simulink model "gm_UZ_EnDat"  (R2023b)
settings: Solver=FixedStepDiscrete  StartTime=0  StopTime=0.002  RelTol=1e-3
model workspace (MAT data in the model file):
  Select = 0
libraries: hdlsllib x314, hdlmdlgenlib x10, simulink x7, simulink_extras x3
(part 5 of 7)

== system gm_UZ_EnDat/UZ_ENDAT/CLKCNTER_ACT/Positional_Counter/Increment Stored Integer ==
  u : Inport  OutDataTypeStr=uint32
  FixPt Constant : Constant  OutDataTypeStr=uint32  SampleTime=-1
  FixPt Data Type Duplicate : DataTypeDuplicate  DisableCoverage=on  NumInputPorts=3
  FixPt Gateway In : DataTypeConversion  OutDataTypeStr=fixdt(0,32,0)
  FixPt Sum1 : Sum  OutDataTypeStr=uint32  AccumDataTypeStr=uint32
  sigspec : SignalSpecification  OutDataTypeStr=uint32  Dimensions=1
  y : Outport  InitialOutput=0
  wires:
  sigspec/1 -> FixPt Gateway In/1
  FixPt Sum1/1 -> y/1, FixPt Data Type Duplicate/1
  FixPt Gateway In/1 -> FixPt Data Type Duplicate/3, FixPt Sum1/2
  FixPt Constant/1 -> sigspec/1
  u/1 -> FixPt Data Type Duplicate/2, FixPt Sum1/1

== system gm_UZ_EnDat/UZ_ENDAT/CLKCNTER_NOSTOP/Positional_Counter/Increment Stored Integer ==
  u : Inport  OutDataTypeStr=uint32
  FixPt Constant : Constant  OutDataTypeStr=uint32  SampleTime=-1
  FixPt Data Type Duplicate : DataTypeDuplicate  DisableCoverage=on  NumInputPorts=3
  FixPt Gateway In : DataTypeConversion  OutDataTypeStr=fixdt(0,32,0)
  FixPt Sum1 : Sum  OutDataTypeStr=uint32  AccumDataTypeStr=uint32
  sigspec : SignalSpecification  OutDataTypeStr=uint32  Dimensions=1
  y : Outport  InitialOutput=0
  wires:
  u/1 -> FixPt Sum1/1, FixPt Data Type Duplicate/2
  FixPt Constant/1 -> sigspec/1
  FixPt Gateway In/1 -> FixPt Sum1/2, FixPt Data Type Duplicate/3
  FixPt Sum1/1 -> FixPt Data Type Duplicate/1, y/1
  sigspec/1 -> FixPt Gateway In/1

== system gm_UZ_EnDat/UZ_ENDAT/CRC_Check/DFF1/JKFF ==
  SET : Inport  OutDataTypeStr=boolean  PortDimensions=1  SampleTime=1e-08
  CLK : Inport  Port=2  OutDataTypeStr=boolean  PortDimensions=1  SampleTime=1e-08
  J : Inport  Port=3  OutDataTypeStr=boolean  PortDimensions=1  SampleTime=1e-08
  RST : Inport  Port=4  OutDataTypeStr=boolean  PortDimensions=1  SampleTime=1e-08
  K : Inport  Port=5  OutDataTypeStr=boolean  PortDimensions=1  SampleTime=1e-08
  AND : Logic  Inputs=4  AllPortsSameDT=off  OutDataTypeStr=boolean  SampleTime=1e-08
  AND1 : Logic  Inputs=4  AllPortsSameDT=off  OutDataTypeStr=boolean  SampleTime=1e-08
  AND{2..5} (4 alike) : Logic  AllPortsSameDT=off  OutDataTypeStr=boolean  SampleTime=1e-08
  Delay{,1..3} (4 alike) : Delay  DelayLength=double(1)  InitialCondition=0  SampleTime=1e-08
  NOR : Logic  Operator=NOR  Inputs=4  AllPortsSameDT=off  OutDataTypeStr=boolean  SampleTime=1e-08
  NOR1 : Logic  Operator=NOR  Inputs=4  AllPortsSameDT=off  OutDataTypeStr=boolean  SampleTime=1e-08
  NOR2 : Logic  Operator=NOR  AllPortsSameDT=off  OutDataTypeStr=boolean  SampleTime=1e-08
  NOR3 : Logic  Operator=NAND  AllPortsSameDT=off  OutDataTypeStr=boolean  SampleTime=1e-08
  NOR4 : Logic  Operator=NOR  AllPortsSameDT=off  OutDataTypeStr=boolean  SampleTime=1e-08
  NOR5 : Logic  Operator=NAND  AllPortsSameDT=off  OutDataTypeStr=boolean  SampleTime=1e-08
  NOT : Logic  Operator=NOT  Inputs=1  AllPortsSameDT=off  OutDataTypeStr=boolean  SampleTime=1e-08
  NOT1 : Logic  Operator=NOT  Inputs=1  AllPortsSameDT=off  OutDataTypeStr=boolean  SampleTime=1e-08
  OR : Logic  Operator=OR  Inputs=3  AllPortsSameDT=off  OutDataTypeStr=boolean  SampleTime=1e-08
  OQ : Outport  SampleTime=1e-08
  NOQ : Outport  Port=2  SampleTime=1e-08
  wires:
  SET/1 -> NOR2/1, NOR/1
  CLK/1 -> OR/2, NOT/1, AND5/1, AND4/2
  J/1 -> OR/1, AND/2
  RST/1 -> NOR1/4, NOR4/2
  K/1 -> OR/3, AND1/3
  Delay2/1 -> NOQ/1, AND2/2, NOR3/2, AND/1
  Delay3/1 -> OQ/1, AND1/4, AND3/1, NOR5/1
  NOT/1 -> AND1/2, AND/3
  NOT1/1 -> AND2/1, AND3/2
  OR/1 -> NOT1/1, AND1/1, AND/4
  Delay/1 -> NOR1/1, AND4/1
  Delay1/1 -> AND5/2, NOR/4
  NOR/1 -> Delay/1
  AND3/1 -> NOR/3
  AND/1 -> NOR/2
  NOR5/1 -> Delay2/1
  AND4/1 -> NOR4/1
  NOR4/1 -> NOR5/2
  NOR1/1 -> Delay1/1
  AND1/1 -> NOR1/3
  AND2/1 -> NOR1/2
  NOR3/1 -> Delay3/1
  AND5/1 -> NOR2/2
  NOR2/1 -> NOR3/1

== system gm_UZ_EnDat/UZ_ENDAT/CRC_Check/DFF2/JKFF ==
  SET : Inport  OutDataTypeStr=boolean  PortDimensions=1  SampleTime=1e-08
  CLK : Inport  Port=2  OutDataTypeStr=boolean  PortDimensions=1  SampleTime=1e-08
  J : Inport  Port=3  OutDataTypeStr=boolean  PortDimensions=1  SampleTime=1e-08
  RST : Inport  Port=4  OutDataTypeStr=boolean  PortDimensions=1  SampleTime=1e-08
  K : Inport  Port=5  OutDataTypeStr=boolean  PortDimensions=1  SampleTime=1e-08
  AND : Logic  Inputs=4  AllPortsSameDT=off  OutDataTypeStr=boolean  SampleTime=1e-08
  AND1 : Logic  Inputs=4  AllPortsSameDT=off  OutDataTypeStr=boolean  SampleTime=1e-08
  AND{2..5} (4 alike) : Logic  AllPortsSameDT=off  OutDataTypeStr=boolean  SampleTime=1e-08
  Delay{,1..3} (4 alike) : Delay  DelayLength=double(1)  InitialCondition=0  SampleTime=1e-08
  NOR : Logic  Operator=NOR  Inputs=4  AllPortsSameDT=off  OutDataTypeStr=boolean  SampleTime=1e-08
  NOR1 : Logic  Operator=NOR  Inputs=4  AllPortsSameDT=off  OutDataTypeStr=boolean  SampleTime=1e-08
  NOR2 : Logic  Operator=NOR  AllPortsSameDT=off  OutDataTypeStr=boolean  SampleTime=1e-08
  NOR3 : Logic  Operator=NAND  AllPortsSameDT=off  OutDataTypeStr=boolean  SampleTime=1e-08
  NOR4 : Logic  Operator=NOR  AllPortsSameDT=off  OutDataTypeStr=boolean  SampleTime=1e-08
  NOR5 : Logic  Operator=NAND  AllPortsSameDT=off  OutDataTypeStr=boolean  SampleTime=1e-08
  NOT : Logic  Operator=NOT  Inputs=1  AllPortsSameDT=off  OutDataTypeStr=boolean  SampleTime=1e-08
  NOT1 : Logic  Operator=NOT  Inputs=1  AllPortsSameDT=off  OutDataTypeStr=boolean  SampleTime=1e-08
  OR : Logic  Operator=OR  Inputs=3  AllPortsSameDT=off  OutDataTypeStr=boolean  SampleTime=1e-08
  OQ : Outport  SampleTime=1e-08
  NOQ : Outport  Port=2  SampleTime=1e-08
  wires:
  NOR2/1 -> NOR3/1
  AND5/1 -> NOR2/2
  NOR3/1 -> Delay3/1
  AND2/1 -> NOR1/2
  AND1/1 -> NOR1/3
  NOR1/1 -> Delay1/1
  NOR4/1 -> NOR5/2
  AND4/1 -> NOR4/1
  NOR5/1 -> Delay2/1
  AND/1 -> NOR/2
  AND3/1 -> NOR/3
  NOR/1 -> Delay/1
  Delay1/1 -> NOR/4, AND5/2
  Delay/1 -> AND4/1, NOR1/1
  OR/1 -> AND/4, AND1/1, NOT1/1
  NOT1/1 -> AND3/2, AND2/1
  NOT/1 -> AND/3, AND1/2
  Delay3/1 -> NOR5/1, AND3/1, AND1/4, OQ/1
  Delay2/1 -> AND/1, NOR3/2, AND2/2, NOQ/1
  K/1 -> AND1/3, OR/3
  RST/1 -> NOR4/2, NOR1/4
  J/1 -> AND/2, OR/1
  CLK/1 -> AND4/2, AND5/1, NOT/1, OR/2
  SET/1 -> NOR/1, NOR2/1

== system gm_UZ_EnDat/UZ_ENDAT/CRC_Check/DFF3/JKFF ==
  SET : Inport  OutDataTypeStr=boolean  PortDimensions=1  SampleTime=1e-08
  CLK : Inport  Port=2  OutDataTypeStr=boolean  PortDimensions=1  SampleTime=1e-08
  J : Inport  Port=3  OutDataTypeStr=boolean  PortDimensions=1  SampleTime=1e-08
  RST : Inport  Port=4  OutDataTypeStr=boolean  PortDimensions=1  SampleTime=1e-08
  K : Inport  Port=5  OutDataTypeStr=boolean  PortDimensions=1  SampleTime=1e-08
  AND : Logic  Inputs=4  AllPortsSameDT=off  OutDataTypeStr=boolean  SampleTime=1e-08
  AND1 : Logic  Inputs=4  AllPortsSameDT=off  OutDataTypeStr=boolean  SampleTime=1e-08
  AND{2..5} (4 alike) : Logic  AllPortsSameDT=off  OutDataTypeStr=boolean  SampleTime=1e-08
  Delay{,1..3} (4 alike) : Delay  DelayLength=double(1)  InitialCondition=0  SampleTime=1e-08
  NOR : Logic  Operator=NOR  Inputs=4  AllPortsSameDT=off  OutDataTypeStr=boolean  SampleTime=1e-08
  NOR1 : Logic  Operator=NOR  Inputs=4  AllPortsSameDT=off  OutDataTypeStr=boolean  SampleTime=1e-08
  NOR2 : Logic  Operator=NOR  AllPortsSameDT=off  OutDataTypeStr=boolean  SampleTime=1e-08
  NOR3 : Logic  Operator=NAND  AllPortsSameDT=off  OutDataTypeStr=boolean  SampleTime=1e-08
  NOR4 : Logic  Operator=NOR  AllPortsSameDT=off  OutDataTypeStr=boolean  SampleTime=1e-08
  NOR5 : Logic  Operator=NAND  AllPortsSameDT=off  OutDataTypeStr=boolean  SampleTime=1e-08
  NOT : Logic  Operator=NOT  Inputs=1  AllPortsSameDT=off  OutDataTypeStr=boolean  SampleTime=1e-08
  NOT1 : Logic  Operator=NOT  Inputs=1  AllPortsSameDT=off  OutDataTypeStr=boolean  SampleTime=1e-08
  OR : Logic  Operator=OR  Inputs=3  AllPortsSameDT=off  OutDataTypeStr=boolean  SampleTime=1e-08
  OQ : Outport  SampleTime=1e-08
  NOQ : Outport  Port=2  SampleTime=1e-08
  wires:
  NOR2/1 -> NOR3/1
  AND5/1 -> NOR2/2
  NOR3/1 -> Delay3/1
  AND2/1 -> NOR1/2
  AND1/1 -> NOR1/3
  NOR1/1 -> Delay1/1
  NOR4/1 -> NOR5/2
  AND4/1 -> NOR4/1
  NOR5/1 -> Delay2/1
  AND/1 -> NOR/2
  AND3/1 -> NOR/3
  NOR/1 -> Delay/1
  Delay1/1 -> NOR/4, AND5/2
  Delay/1 -> AND4/1, NOR1/1
  OR/1 -> AND/4, AND1/1, NOT1/1
  NOT1/1 -> AND3/2, AND2/1
  NOT/1 -> AND/3, AND1/2
  Delay3/1 -> NOR5/1, AND3/1, AND1/4, OQ/1
  Delay2/1 -> AND/1, NOR3/2, AND2/2, NOQ/1
  K/1 -> AND1/3, OR/3
  RST/1 -> NOR4/2, NOR1/4
  J/1 -> AND/2, OR/1
  CLK/1 -> AND4/2, AND5/1, NOT/1, OR/2
  SET/1 -> NOR/1, NOR2/1

== system gm_UZ_EnDat/UZ_ENDAT/CRC_Check/DFF4/JKFF ==
  SET : Inport  OutDataTypeStr=boolean  PortDimensions=1  SampleTime=1e-08
  CLK : Inport  Port=2  OutDataTypeStr=boolean  PortDimensions=1  SampleTime=1e-08
  J : Inport  Port=3  OutDataTypeStr=boolean  PortDimensions=1  SampleTime=1e-08
  RST : Inport  Port=4  OutDataTypeStr=boolean  PortDimensions=1  SampleTime=1e-08
  K : Inport  Port=5  OutDataTypeStr=boolean  PortDimensions=1  SampleTime=1e-08
  AND : Logic  Inputs=4  AllPortsSameDT=off  OutDataTypeStr=boolean  SampleTime=1e-08
  AND1 : Logic  Inputs=4  AllPortsSameDT=off  OutDataTypeStr=boolean  SampleTime=1e-08
  AND{2..5} (4 alike) : Logic  AllPortsSameDT=off  OutDataTypeStr=boolean  SampleTime=1e-08
  Delay{,1..3} (4 alike) : Delay  DelayLength=double(1)  InitialCondition=0  SampleTime=1e-08
  NOR : Logic  Operator=NOR  Inputs=4  AllPortsSameDT=off  OutDataTypeStr=boolean  SampleTime=1e-08
  NOR1 : Logic  Operator=NOR  Inputs=4  AllPortsSameDT=off  OutDataTypeStr=boolean  SampleTime=1e-08
  NOR2 : Logic  Operator=NOR  AllPortsSameDT=off  OutDataTypeStr=boolean  SampleTime=1e-08
  NOR3 : Logic  Operator=NAND  AllPortsSameDT=off  OutDataTypeStr=boolean  SampleTime=1e-08
  NOR4 : Logic  Operator=NOR  AllPortsSameDT=off  OutDataTypeStr=boolean  SampleTime=1e-08
  NOR5 : Logic  Operator=NAND  AllPortsSameDT=off  OutDataTypeStr=boolean  SampleTime=1e-08
  NOT : Logic  Operator=NOT  Inputs=1  AllPortsSameDT=off  OutDataTypeStr=boolean  SampleTime=1e-08
  NOT1 : Logic  Operator=NOT  Inputs=1  AllPortsSameDT=off  OutDataTypeStr=boolean  SampleTime=1e-08
  OR : Logic  Operator=OR  Inputs=3  AllPortsSameDT=off  OutDataTypeStr=boolean  SampleTime=1e-08
  OQ : Outport  SampleTime=1e-08
  NOQ : Outport  Port=2  SampleTime=1e-08
  wires:
  NOR2/1 -> NOR3/1
  AND5/1 -> NOR2/2
  NOR3/1 -> Delay3/1
  AND2/1 -> NOR1/2
  AND1/1 -> NOR1/3
  NOR1/1 -> Delay1/1
  NOR4/1 -> NOR5/2
  AND4/1 -> NOR4/1
  NOR5/1 -> Delay2/1
  AND/1 -> NOR/2
  AND3/1 -> NOR/3
  NOR/1 -> Delay/1
  Delay1/1 -> NOR/4, AND5/2
  Delay/1 -> AND4/1, NOR1/1
  OR/1 -> AND/4, AND1/1, NOT1/1
  NOT1/1 -> AND3/2, AND2/1
  NOT/1 -> AND/3, AND1/2
  Delay3/1 -> NOR5/1, AND3/1, AND1/4, OQ/1
  Delay2/1 -> AND/1, NOR3/2, AND2/2, NOQ/1
  K/1 -> AND1/3, OR/3
  RST/1 -> NOR4/2, NOR1/4
  J/1 -> AND/2, OR/1
  CLK/1 -> AND4/2, AND5/1, NOT/1, OR/2
  SET/1 -> NOR/1, NOR2/1

== system gm_UZ_EnDat/UZ_ENDAT/CRC_Check/DFF5/JKFF ==
  SET : Inport  OutDataTypeStr=boolean  PortDimensions=1  SampleTime=1e-08
  CLK : Inport  Port=2  OutDataTypeStr=boolean  PortDimensions=1  SampleTime=1e-08
  J : Inport  Port=3  OutDataTypeStr=boolean  PortDimensions=1  SampleTime=1e-08
  RST : Inport  Port=4  OutDataTypeStr=boolean  PortDimensions=1  SampleTime=1e-08
  K : Inport  Port=5  OutDataTypeStr=boolean  PortDimensions=1  SampleTime=1e-08
  AND : Logic  Inputs=4  AllPortsSameDT=off  OutDataTypeStr=boolean  SampleTime=1e-08
  AND1 : Logic  Inputs=4  AllPortsSameDT=off  OutDataTypeStr=boolean  SampleTime=1e-08
  AND{2..5} (4 alike) : Logic  AllPortsSameDT=off  OutDataTypeStr=boolean  SampleTime=1e-08
  Delay{,1..3} (4 alike) : Delay  DelayLength=double(1)  InitialCondition=0  SampleTime=1e-08
  NOR : Logic  Operator=NOR  Inputs=4  AllPortsSameDT=off  OutDataTypeStr=boolean  SampleTime=1e-08
  NOR1 : Logic  Operator=NOR  Inputs=4  AllPortsSameDT=off  OutDataTypeStr=boolean  SampleTime=1e-08
  NOR2 : Logic  Operator=NOR  AllPortsSameDT=off  OutDataTypeStr=boolean  SampleTime=1e-08
  NOR3 : Logic  Operator=NAND  AllPortsSameDT=off  OutDataTypeStr=boolean  SampleTime=1e-08
  NOR4 : Logic  Operator=NOR  AllPortsSameDT=off  OutDataTypeStr=boolean  SampleTime=1e-08
  NOR5 : Logic  Operator=NAND  AllPortsSameDT=off  OutDataTypeStr=boolean  SampleTime=1e-08
  NOT : Logic  Operator=NOT  Inputs=1  AllPortsSameDT=off  OutDataTypeStr=boolean  SampleTime=1e-08
  NOT1 : Logic  Operator=NOT  Inputs=1  AllPortsSameDT=off  OutDataTypeStr=boolean  SampleTime=1e-08
  OR : Logic  Operator=OR  Inputs=3  AllPortsSameDT=off  OutDataTypeStr=boolean  SampleTime=1e-08
  OQ : Outport  SampleTime=1e-08
  NOQ : Outport  Port=2  SampleTime=1e-08
  wires:
  NOR2/1 -> NOR3/1
  AND5/1 -> NOR2/2
  NOR3/1 -> Delay3/1
  AND2/1 -> NOR1/2
  AND1/1 -> NOR1/3
  NOR1/1 -> Delay1/1
  NOR4/1 -> NOR5/2
  AND4/1 -> NOR4/1
  NOR5/1 -> Delay2/1
  AND/1 -> NOR/2
  AND3/1 -> NOR/3
  NOR/1 -> Delay/1
  Delay1/1 -> NOR/4, AND5/2
  Delay/1 -> AND4/1, NOR1/1
  OR/1 -> AND/4, AND1/1, NOT1/1
  NOT1/1 -> AND3/2, AND2/1
  NOT/1 -> AND/3, AND1/2
  Delay3/1 -> NOR5/1, AND3/1, AND1/4, OQ/1
  Delay2/1 -> AND/1, NOR3/2, AND2/2, NOQ/1
  K/1 -> AND1/3, OR/3
  RST/1 -> NOR4/2, NOR1/4
  J/1 -> AND/2, OR/1
  CLK/1 -> AND4/2, AND5/1, NOT/1, OR/2
  SET/1 -> NOR/1, NOR2/1

== system gm_UZ_EnDat/UZ_ENDAT/INITIALOFF/CLKCNTER_FAST/Positional_Counter ==
  valueout : Inport  OutDataTypeStr=uint32  PortDimensions=1
  Trigger : TriggerPort  TriggerType=either  VariantControl=(inherit)  InitialTriggerSignalState=zero  PortDimensions=1  OutDataTypeStr=boolean
  Add : Sum  OutDataTypeStr=fixdt(0, 33, 0)  AccumDataTypeStr=fixdt(0, 33, 0)
  Add_out_dtc : DataTypeConversion  OutDataTypeStr=uint32  RndMeth=Simplest
  Constant : Constant  OutDataTypeStr=uint32  SampleTime=-1
  divider : Outport  InitialOutput=0
  wires:
  valueout/1 -> Add/1
  Add_out_dtc/1 -> divider/1
  Constant/1 -> Add/2
  Add/1 -> Add_out_dtc/1

== system gm_UZ_EnDat/UZ_ENDAT/INITIALOFF/Subsystem6/Compare To Constant ==
  u : Inport  OutDataTypeStr=uint16  SampleTime=1e-08
  Compare : RelationalOperator  Operator=<  OutDataTypeStr=boolean  SampleTime=1e-08
  Constant : Constant  Value=100  OutDataTypeStr=uint16  SampleTime=1e-08
  y : Outport  SampleTime=1e-08
  wires:
  u/1 -> Compare/1
  Compare/1 -> y/1
  Constant/1 -> Compare/2

== system gm_UZ_EnDat/UZ_ENDAT/ManualSerialize/Storage1/Compare To Zero ==
  u : Inport  OutDataTypeStr=fixdt(0, 64, 0)  SampleTime=1e-08
  Compare : RelationalOperator  Operator=>  OutDataTypeStr=boolean  SampleTime=1e-08
  Constant : Constant  Value="fi(0,0,64,0,\"hex\",\"0000000000000000\")"  OutDataTypeStr=fixdt(0, 64, 0)  SampleTime=1e-08
  y : Outport  SampleTime=1e-08
  wires:
  u/1 -> Compare/1
  Compare/1 -> y/1
  Constant/1 -> Compare/2

== system gm_UZ_EnDat/UZ_ENDAT/ManualSerialize/Subsystem/Detect Increase ==
  note: U(k)
  note: Edge
  U : Inport  OutDataTypeStr=boolean  SampleTime=1e-08
  FixPt Relational Operator : RelationalOperator  Operator=>  OutDataTypeStr=boolean  SampleTime=1e-08  InputSameDT=off
  rd_0 : Delay  DelayLength=double(1)  InitialCondition=0  SampleTime=1e-08
  t : hdlmdlgenlib/Buffer
  Y : Outport  SampleTime=1e-08
  wires:
  U/1 -> t/1, FixPt Relational Operator/1
  t/1 -> rd_0/1
  FixPt Relational Operator/1 -> Y/1
  rd_0/1 -> FixPt Relational Operator/2

== system gm_UZ_EnDat/UZ_ENDAT/ManualSerialize/padder/nibblepadding1 ==
  in : Inport  OutDataTypeStr=fixdt(0, 64, 0)  PortDimensions=1  SampleTime=1e-08
  padding1 : Subsystem
  padding2 : Subsystem
  padding3 : Subsystem
  out : Outport  SampleTime=1e-08
  wires:
  in/1 -> padding3/1(in)
  padding1/1(out) -> out/1
  padding2/1(out) -> padding1/1(in)
  padding3/1(out) -> padding2/1(in)

== system gm_UZ_EnDat/UZ_ENDAT/ManualSerialize/padder/nibblepadding10 ==
  in : Inport  OutDataTypeStr=fixdt(0, 64, 0)  PortDimensions=1  SampleTime=1e-08
  padding1 : Subsystem
  padding2 : Subsystem
  padding3 : Subsystem
  out : Outport  SampleTime=1e-08
  wires:
  padding3/1(out) -> padding2/1(in)
  padding2/1(out) -> padding1/1(in)
  padding1/1(out) -> out/1
  in/1 -> padding3/1(in)

== system gm_UZ_EnDat/UZ_ENDAT/ManualSerialize/padder/nibblepadding11 ==
  in : Inport  OutDataTypeStr=fixdt(0, 64, 0)  PortDimensions=1  SampleTime=1e-08
  padding1 : Subsystem
  padding2 : Subsystem
  padding3 : Subsystem
  out : Outport  SampleTime=1e-08
  wires:
  padding3/1(out) -> padding2/1(in)
  padding2/1(out) -> padding1/1(in)
  padding1/1(out) -> out/1
  in/1 -> padding3/1(in)

== system gm_UZ_EnDat/UZ_ENDAT/ManualSerialize/padder/nibblepadding12 ==
  in : Inport  OutDataTypeStr=fixdt(0, 64, 0)  PortDimensions=1  SampleTime=1e-08
  padding1 : Subsystem
  padding2 : Subsystem
  padding3 : Subsystem
  out : Outport  SampleTime=1e-08
  wires:
  padding3/1(out) -> padding2/1(in)
  padding2/1(out) -> padding1/1(in)
  padding1/1(out) -> out/1
  in/1 -> padding3/1(in)

== system gm_UZ_EnDat/UZ_ENDAT/ManualSerialize/padder/nibblepadding13 ==
  in : Inport  OutDataTypeStr=fixdt(0, 64, 0)  PortDimensions=1  SampleTime=1e-08
  padding1 : Subsystem
  padding2 : Subsystem
  padding3 : Subsystem
  out : Outport  SampleTime=1e-08
  wires:
  padding3/1(out) -> padding2/1(in)
  padding2/1(out) -> padding1/1(in)
  padding1/1(out) -> out/1
  in/1 -> padding3/1(in)

== system gm_UZ_EnDat/UZ_ENDAT/ManualSerialize/padder/nibblepadding14 ==
  in : Inport  OutDataTypeStr=fixdt(0, 64, 0)  PortDimensions=1  SampleTime=1e-08
  padding1 : Subsystem
  padding2 : Subsystem
  padding3 : Subsystem
  out : Outport  SampleTime=1e-08
  wires:
  padding3/1(out) -> padding2/1(in)
  padding2/1(out) -> padding1/1(in)
  padding1/1(out) -> out/1
  in/1 -> padding3/1(in)

== system gm_UZ_EnDat/UZ_ENDAT/ManualSerialize/padder/nibblepadding15 ==
  in : Inport  OutDataTypeStr=fixdt(0, 64, 0)  PortDimensions=1  SampleTime=1e-08
  padding1 : Subsystem
  padding2 : Subsystem
  padding3 : Subsystem
  out : Outport  SampleTime=1e-08
  wires:
  padding3/1(out) -> padding2/1(in)
  padding2/1(out) -> padding1/1(in)
  padding1/1(out) -> out/1
  in/1 -> padding3/1(in)

== system gm_UZ_EnDat/UZ_ENDAT/ManualSerialize/padder/nibblepadding16 ==
  in : Inport  OutDataTypeStr=fixdt(0, 64, 0)  PortDimensions=1  SampleTime=1e-08
  padding1 : Subsystem
  padding2 : Subsystem
  padding3 : Subsystem
  out : Outport  SampleTime=1e-08
  wires:
  padding3/1(out) -> padding2/1(in)
  padding2/1(out) -> padding1/1(in)
  padding1/1(out) -> out/1
  in/1 -> padding3/1(in)

== system gm_UZ_EnDat/UZ_ENDAT/ManualSerialize/padder/nibblepadding17 ==
  in : Inport  OutDataTypeStr=fixdt(0, 64, 0)  PortDimensions=1  SampleTime=1e-08
  padding1 : Subsystem
  padding2 : Subsystem
  padding3 : Subsystem
  out : Outport  SampleTime=1e-08
  wires:
  padding3/1(out) -> padding2/1(in)
  padding2/1(out) -> padding1/1(in)
  padding1/1(out) -> out/1
  in/1 -> padding3/1(in)

== system gm_UZ_EnDat/UZ_ENDAT/ManualSerialize/padder/nibblepadding18 ==
  in : Inport  OutDataTypeStr=fixdt(0, 64, 0)  PortDimensions=1  SampleTime=1e-08
  padding1 : Subsystem
  padding2 : Subsystem
  padding3 : Subsystem
  out : Outport  SampleTime=1e-08
  wires:
  padding3/1(out) -> padding2/1(in)
  padding2/1(out) -> padding1/1(in)
  padding1/1(out) -> out/1
  in/1 -> padding3/1(in)

== system gm_UZ_EnDat/UZ_ENDAT/ManualSerialize/padder/nibblepadding19 ==
  in : Inport  OutDataTypeStr=fixdt(0, 64, 0)  PortDimensions=1  SampleTime=1e-08
  padding1 : Subsystem
  padding2 : Subsystem
  padding3 : Subsystem
  out : Outport  SampleTime=1e-08
  wires:
  padding3/1(out) -> padding2/1(in)
  padding2/1(out) -> padding1/1(in)
  padding1/1(out) -> out/1
  in/1 -> padding3/1(in)

== system gm_UZ_EnDat/UZ_ENDAT/ManualSerialize/padder/nibblepadding2 ==
  in : Inport  OutDataTypeStr=fixdt(0, 64, 0)  PortDimensions=1  SampleTime=1e-08
  padding1 : Subsystem
  padding2 : Subsystem
  padding3 : Subsystem
  out : Outport  SampleTime=1e-08
  wires:
  padding3/1(out) -> padding2/1(in)
  padding2/1(out) -> padding1/1(in)
  padding1/1(out) -> out/1
  in/1 -> padding3/1(in)

== system gm_UZ_EnDat/UZ_ENDAT/ManualSerialize/padder/nibblepadding20 ==
  in : Inport  OutDataTypeStr=fixdt(0, 64, 0)  PortDimensions=1  SampleTime=1e-08
  padding1 : Subsystem
  padding2 : Subsystem
  padding3 : Subsystem
  out : Outport  SampleTime=1e-08
  wires:
  padding3/1(out) -> padding2/1(in)
  padding2/1(out) -> padding1/1(in)
  padding1/1(out) -> out/1
  in/1 -> padding3/1(in)

== system gm_UZ_EnDat/UZ_ENDAT/ManualSerialize/padder/nibblepadding21 ==
  in : Inport  OutDataTypeStr=fixdt(0, 64, 0)  PortDimensions=1  SampleTime=1e-08
  padding1 : Subsystem
  padding2 : Subsystem
  padding3 : Subsystem
  out : Outport  SampleTime=1e-08
  wires:
  padding3/1(out) -> padding2/1(in)
  padding2/1(out) -> padding1/1(in)
  padding1/1(out) -> out/1
  in/1 -> padding3/1(in)

== system gm_UZ_EnDat/UZ_ENDAT/ManualSerialize/padder/nibblepadding22 ==
  in : Inport  OutDataTypeStr=fixdt(0, 64, 0)  PortDimensions=1  SampleTime=1e-08
  padding1 : Subsystem
  padding2 : Subsystem
  padding3 : Subsystem
  out : Outport  SampleTime=1e-08
  wires:
  padding3/1(out) -> padding2/1(in)
  padding2/1(out) -> padding1/1(in)
  padding1/1(out) -> out/1
  in/1 -> padding3/1(in)

== system gm_UZ_EnDat/UZ_ENDAT/ManualSerialize/padder/nibblepadding23 ==
  in : Inport  OutDataTypeStr=fixdt(0, 64, 0)  PortDimensions=1  SampleTime=1e-08
  padding1 : Subsystem
  padding2 : Subsystem
  padding3 : Subsystem
  out : Outport  SampleTime=1e-08
  wires:
  padding3/1(out) -> padding2/1(in)
  padding2/1(out) -> padding1/1(in)
  padding1/1(out) -> out/1
  in/1 -> padding3/1(in)

== system gm_UZ_EnDat/UZ_ENDAT/ManualSerialize/padder/nibblepadding24 ==
  in : Inport  OutDataTypeStr=fixdt(0, 64, 0)  PortDimensions=1  SampleTime=1e-08
  padding1 : Subsystem
  padding2 : Subsystem
  padding3 : Subsystem
  out : Outport  SampleTime=1e-08
  wires:
  padding3/1(out) -> padding2/1(in)
  padding2/1(out) -> padding1/1(in)
  padding1/1(out) -> out/1
  in/1 -> padding3/1(in)

== system gm_UZ_EnDat/UZ_ENDAT/ManualSerialize/padder/nibblepadding25 ==
  in : Inport  OutDataTypeStr=fixdt(0, 64, 0)  PortDimensions=1  SampleTime=1e-08
  padding1 : Subsystem
  padding2 : Subsystem
  padding3 : Subsystem
  out : Outport  SampleTime=1e-08
  wires:
  padding3/1(out) -> padding2/1(in)
  padding2/1(out) -> padding1/1(in)
  padding1/1(out) -> out/1
  in/1 -> padding3/1(in)

== system gm_UZ_EnDat/UZ_ENDAT/ManualSerialize/padder/nibblepadding26 ==
  in : Inport  OutDataTypeStr=fixdt(0, 64, 0)  PortDimensions=1  SampleTime=1e-08
  padding1 : Subsystem
  padding2 : Subsystem
  padding3 : Subsystem
  out : Outport  SampleTime=1e-08
  wires:
  padding3/1(out) -> padding2/1(in)
  padding2/1(out) -> padding1/1(in)
  padding1/1(out) -> out/1
  in/1 -> padding3/1(in)

== system gm_UZ_EnDat/UZ_ENDAT/ManualSerialize/padder/nibblepadding27 ==
  in : Inport  OutDataTypeStr=fixdt(0, 64, 0)  PortDimensions=1  SampleTime=1e-08
  padding1 : Subsystem
  padding2 : Subsystem
  padding3 : Subsystem
  out : Outport  SampleTime=1e-08
  wires:
  padding3/1(out) -> padding2/1(in)
  padding2/1(out) -> padding1/1(in)
  padding1/1(out) -> out/1
  in/1 -> padding3/1(in)

== system gm_UZ_EnDat/UZ_ENDAT/ManualSerialize/padder/nibblepadding28 ==
  in : Inport  OutDataTypeStr=fixdt(0, 64, 0)  PortDimensions=1  SampleTime=1e-08
  padding1 : Subsystem
  padding2 : Subsystem
  padding3 : Subsystem
  out : Outport  SampleTime=1e-08
  wires:
  padding3/1(out) -> padding2/1(in)
  padding2/1(out) -> padding1/1(in)
  padding1/1(out) -> out/1
  in/1 -> padding3/1(in)

== system gm_UZ_EnDat/UZ_ENDAT/ManualSerialize/padder/nibblepadding29 ==
  in : Inport  OutDataTypeStr=fixdt(0, 64, 0)  PortDimensions=1  SampleTime=1e-08
  padding1 : Subsystem
  padding2 : Subsystem
  padding3 : Subsystem
  out : Outport  SampleTime=1e-08
  wires:
  padding3/1(out) -> padding2/1(in)
  padding2/1(out) -> padding1/1(in)
  padding1/1(out) -> out/1
  in/1 -> padding3/1(in)

== system gm_UZ_EnDat/UZ_ENDAT/ManualSerialize/padder/nibblepadding3 ==
  in : Inport  OutDataTypeStr=fixdt(0, 64, 0)  PortDimensions=1  SampleTime=1e-08
  padding1 : Subsystem
  padding2 : Subsystem
  padding3 : Subsystem
  out : Outport  SampleTime=1e-08
  wires:
  padding3/1(out) -> padding2/1(in)
  padding2/1(out) -> padding1/1(in)
  padding1/1(out) -> out/1
  in/1 -> padding3/1(in)

== system gm_UZ_EnDat/UZ_ENDAT/ManualSerialize/padder/nibblepadding30 ==
  in : Inport  OutDataTypeStr=fixdt(0, 64, 0)  PortDimensions=1  SampleTime=1e-08
  padding1 : Subsystem
  padding2 : Subsystem
  padding3 : Subsystem
  out : Outport  SampleTime=1e-08
  wires:
  padding3/1(out) -> padding2/1(in)
  padding2/1(out) -> padding1/1(in)
  padding1/1(out) -> out/1
  in/1 -> padding3/1(in)

== system gm_UZ_EnDat/UZ_ENDAT/ManualSerialize/padder/nibblepadding4 ==
  in : Inport  OutDataTypeStr=fixdt(0, 64, 0)  PortDimensions=1  SampleTime=1e-08
  padding1 : Subsystem
  padding2 : Subsystem
  padding3 : Subsystem
  out : Outport  SampleTime=1e-08
  wires:
  padding3/1(out) -> padding2/1(in)
  padding2/1(out) -> padding1/1(in)
  padding1/1(out) -> out/1
  in/1 -> padding3/1(in)

== system gm_UZ_EnDat/UZ_ENDAT/ManualSerialize/padder/nibblepadding6 ==
  in : Inport  OutDataTypeStr=fixdt(0, 64, 0)  PortDimensions=1  SampleTime=1e-08
  padding1 : Subsystem
  padding2 : Subsystem
  padding3 : Subsystem
  out : Outport  SampleTime=1e-08
  wires:
  padding3/1(out) -> padding2/1(in)
  padding2/1(out) -> padding1/1(in)
  padding1/1(out) -> out/1
  in/1 -> padding3/1(in)

== system gm_UZ_EnDat/UZ_ENDAT/ManualSerialize/padder/nibblepadding7 ==
  in : Inport  OutDataTypeStr=fixdt(0, 64, 0)  PortDimensions=1  SampleTime=1e-08
  padding1 : Subsystem
  padding2 : Subsystem
  padding3 : Subsystem
  out : Outport  SampleTime=1e-08
  wires:
  padding3/1(out) -> padding2/1(in)
  padding2/1(out) -> padding1/1(in)
  padding1/1(out) -> out/1
  in/1 -> padding3/1(in)

== system gm_UZ_EnDat/UZ_ENDAT/ManualSerialize/padder/nibblepadding8 ==
  in : Inport  OutDataTypeStr=fixdt(0, 64, 0)  PortDimensions=1  SampleTime=1e-08
  padding1 : Subsystem
  padding2 : Subsystem
  padding3 : Subsystem
  out : Outport  SampleTime=1e-08
  wires:
  padding3/1(out) -> padding2/1(in)
  padding2/1(out) -> padding1/1(in)
  padding1/1(out) -> out/1
  in/1 -> padding3/1(in)

== system gm_UZ_EnDat/UZ_ENDAT/ManualSerialize/padder/nibblepadding9 ==
  in : Inport  OutDataTypeStr=fixdt(0, 64, 0)  PortDimensions=1  SampleTime=1e-08
  padding1 : Subsystem
  padding2 : Subsystem
  padding3 : Subsystem
  out : Outport  SampleTime=1e-08
  wires:
  padding3/1(out) -> padding2/1(in)
  padding2/1(out) -> padding1/1(in)
  padding1/1(out) -> out/1
  in/1 -> padding3/1(in)

== system gm_UZ_EnDat/UZ_ENDAT/RESPONSESLICER3X/19BITSLICER/responseslicer ==
  DATA : Inport  OutDataTypeStr=fixdt(0, 64, 0)  PortDimensions=1  SampleTime=1e-08
  Bit Slice1 : hdlsllib/Logic and Bit Operations/Bit Slice  lidx=double(2)  ridx=double(2)
  Bit Slice3 : hdlsllib/Logic and Bit Operations/Bit Slice  lidx=double(25)  ridx=double(21)
  Bit Slice4 : hdlsllib/Logic and Bit Operations/Bit Slice  lidx=double(20)  ridx=double(2)
  Data Type Conversion1 : DataTypeConversion  OutDataTypeStr=boolean  SampleTime=1e-08  SaturateOnIntegerOverflow=off  RndMeth=Floor
  Data Type Conversion3 : DataTypeConversion  OutDataTypeStr=uint8  SampleTime=1e-08  SaturateOnIntegerOverflow=off  RndMeth=Floor
  Data Type Conversion4 : DataTypeConversion  OutDataTypeStr=uint32  SampleTime=1e-08  SaturateOnIntegerOverflow=off  RndMeth=Floor
  CRC : Outport  OutDataTypeStr=uint8  SampleTime=1e-08  InitialOutput=0
  payload : Outport  Port=2  OutDataTypeStr=uint32  SampleTime=1e-08  InitialOutput=0
  error : Outport  Port=3  OutDataTypeStr=boolean  SampleTime=1e-08  InitialOutput=0
  wires:
  DATA/1 -> Bit Slice4/1, Bit Slice3/1, Bit Slice1/1
  Bit Slice1/1 -> Data Type Conversion1/1
  Bit Slice3/1 -> Data Type Conversion3/1
  Bit Slice4/1 -> Data Type Conversion4/1
  Data Type Conversion1/1 -> error/1
  Data Type Conversion3/1 -> CRC/1
  Data Type Conversion4/1 -> payload/1

== system gm_UZ_EnDat/UZ_ENDAT/RESPONSESLICER3X/19BITSLICER/responseslicer1 ==
  DATA : Inport  OutDataTypeStr=fixdt(0, 64, 0)  PortDimensions=1  SampleTime=1e-08
  Bit Slice1 : hdlsllib/Logic and Bit Operations/Bit Slice  lidx=double(2)  ridx=double(2)
  Bit Slice3 : hdlsllib/Logic and Bit Operations/Bit Slice  lidx=double(25)  ridx=double(21)
  Bit Slice4 : hdlsllib/Logic and Bit Operations/Bit Slice  lidx=double(20)  ridx=double(2)
  Data Type Conversion1 : DataTypeConversion  OutDataTypeStr=boolean  SampleTime=1e-08  SaturateOnIntegerOverflow=off  RndMeth=Floor
  Data Type Conversion3 : DataTypeConversion  OutDataTypeStr=uint8  SampleTime=1e-08  SaturateOnIntegerOverflow=off  RndMeth=Floor
  Data Type Conversion4 : DataTypeConversion  OutDataTypeStr=uint32  SampleTime=1e-08  SaturateOnIntegerOverflow=off  RndMeth=Floor
  CRC : Outport  OutDataTypeStr=uint8  SampleTime=1e-08  InitialOutput=0
  payload : Outport  Port=2  OutDataTypeStr=uint32  SampleTime=1e-08  InitialOutput=0
  error : Outport  Port=3  OutDataTypeStr=boolean  SampleTime=1e-08  InitialOutput=0
  wires:
  Data Type Conversion4/1 -> payload/1
  Data Type Conversion3/1 -> CRC/1
  Data Type Conversion1/1 -> error/1
  Bit Slice4/1 -> Data Type Conversion4/1
  Bit Slice3/1 -> Data Type Conversion3/1
  Bit Slice1/1 -> Data Type Conversion1/1
  DATA/1 -> Bit Slice1/1, Bit Slice3/1, Bit Slice4/1

== system gm_UZ_EnDat/UZ_ENDAT/RESPONSESLICER3X/19BITSLICER/responseslicer2 ==
  DATA : Inport  OutDataTypeStr=fixdt(0, 64, 0)  PortDimensions=1  SampleTime=1e-08
  Bit Slice1 : hdlsllib/Logic and Bit Operations/Bit Slice  lidx=double(2)  ridx=double(2)
  Bit Slice3 : hdlsllib/Logic and Bit Operations/Bit Slice  lidx=double(25)  ridx=double(21)
  Bit Slice4 : hdlsllib/Logic and Bit Operations/Bit Slice  lidx=double(20)  ridx=double(2)
  Data Type Conversion1 : DataTypeConversion  OutDataTypeStr=boolean  SampleTime=1e-08  SaturateOnIntegerOverflow=off  RndMeth=Floor
  Data Type Conversion3 : DataTypeConversion  OutDataTypeStr=uint8  SampleTime=1e-08  SaturateOnIntegerOverflow=off  RndMeth=Floor
  Data Type Conversion4 : DataTypeConversion  OutDataTypeStr=uint32  SampleTime=1e-08  SaturateOnIntegerOverflow=off  RndMeth=Floor
  CRC : Outport  OutDataTypeStr=uint8  SampleTime=1e-08  InitialOutput=0
  payload : Outport  Port=2  OutDataTypeStr=uint32  SampleTime=1e-08  InitialOutput=0
  error : Outport  Port=3  OutDataTypeStr=boolean  SampleTime=1e-08  InitialOutput=0
  wires:
  Data Type Conversion4/1 -> payload/1
  Data Type Conversion3/1 -> CRC/1
  Data Type Conversion1/1 -> error/1
  Bit Slice4/1 -> Data Type Conversion4/1
  Bit Slice3/1 -> Data Type Conversion3/1
  Bit Slice1/1 -> Data Type Conversion1/1
  DATA/1 -> Bit Slice1/1, Bit Slice3/1, Bit Slice4/1

== system gm_UZ_EnDat/UZ_ENDAT/RESPONSESLICER3X/21BITSLICER/responseslicer ==
  DATA : Inport  OutDataTypeStr=fixdt(0, 64, 0)  PortDimensions=1  SampleTime=1e-08
  Bit Slice1 : hdlsllib/Logic and Bit Operations/Bit Slice  lidx=double(2)  ridx=double(2)
  Bit Slice3 : hdlsllib/Logic and Bit Operations/Bit Slice  lidx=double(27)  ridx=double(23)
  Bit Slice4 : hdlsllib/Logic and Bit Operations/Bit Slice  lidx=double(22)  ridx=double(2)
  Data Type Conversion1 : DataTypeConversion  OutDataTypeStr=boolean  SampleTime=1e-08  SaturateOnIntegerOverflow=off  RndMeth=Floor
  Data Type Conversion3 : DataTypeConversion  OutDataTypeStr=uint8  SampleTime=1e-08  SaturateOnIntegerOverflow=off  RndMeth=Floor
  Data Type Conversion4 : DataTypeConversion  OutDataTypeStr=uint32  SampleTime=1e-08  SaturateOnIntegerOverflow=off  RndMeth=Floor
  CRC : Outport  OutDataTypeStr=uint8  SampleTime=1e-08  InitialOutput=0
  payload : Outport  Port=2  OutDataTypeStr=uint32  SampleTime=1e-08  InitialOutput=0
  error : Outport  Port=3  OutDataTypeStr=boolean  SampleTime=1e-08  InitialOutput=0
  wires:
  DATA/1 -> Bit Slice4/1, Bit Slice3/1, Bit Slice1/1
  Bit Slice1/1 -> Data Type Conversion1/1
  Bit Slice3/1 -> Data Type Conversion3/1
  Bit Slice4/1 -> Data Type Conversion4/1
  Data Type Conversion1/1 -> error/1
  Data Type Conversion3/1 -> CRC/1
  Data Type Conversion4/1 -> payload/1

== system gm_UZ_EnDat/UZ_ENDAT/RESPONSESLICER3X/21BITSLICER/responseslicer3 ==
  DATA : Inport  OutDataTypeStr=fixdt(0, 64, 0)  PortDimensions=1  SampleTime=1e-08
  Bit Slice1 : hdlsllib/Logic and Bit Operations/Bit Slice  lidx=double(2)  ridx=double(2)
  Bit Slice3 : hdlsllib/Logic and Bit Operations/Bit Slice  lidx=double(27)  ridx=double(23)
  Bit Slice4 : hdlsllib/Logic and Bit Operations/Bit Slice  lidx=double(22)  ridx=double(2)
  Data Type Conversion1 : DataTypeConversion  OutDataTypeStr=boolean  SampleTime=1e-08  SaturateOnIntegerOverflow=off  RndMeth=Floor
  Data Type Conversion3 : DataTypeConversion  OutDataTypeStr=uint8  SampleTime=1e-08  SaturateOnIntegerOverflow=off  RndMeth=Floor
  Data Type Conversion4 : DataTypeConversion  OutDataTypeStr=uint32  SampleTime=1e-08  SaturateOnIntegerOverflow=off  RndMeth=Floor
  CRC : Outport  OutDataTypeStr=uint8  SampleTime=1e-08  InitialOutput=0
  payload : Outport  Port=2  OutDataTypeStr=uint32  SampleTime=1e-08  InitialOutput=0
  error : Outport  Port=3  OutDataTypeStr=boolean  SampleTime=1e-08  InitialOutput=0
  wires:
  Data Type Conversion4/1 -> payload/1
  Data Type Conversion3/1 -> CRC/1
  Data Type Conversion1/1 -> error/1
  Bit Slice4/1 -> Data Type Conversion4/1
  Bit Slice3/1 -> Data Type Conversion3/1
  Bit Slice1/1 -> Data Type Conversion1/1
  DATA/1 -> Bit Slice1/1, Bit Slice3/1, Bit Slice4/1

== system gm_UZ_EnDat/UZ_ENDAT/RESPONSESLICER3X/21BITSLICER/responseslicer4 ==
  DATA : Inport  OutDataTypeStr=fixdt(0, 64, 0)  PortDimensions=1  SampleTime=1e-08
  Bit Slice1 : hdlsllib/Logic and Bit Operations/Bit Slice  lidx=double(2)  ridx=double(2)
  Bit Slice3 : hdlsllib/Logic and Bit Operations/Bit Slice  lidx=double(27)  ridx=double(23)
  Bit Slice4 : hdlsllib/Logic and Bit Operations/Bit Slice  lidx=double(22)  ridx=double(2)
  Data Type Conversion1 : DataTypeConversion  OutDataTypeStr=boolean  SampleTime=1e-08  SaturateOnIntegerOverflow=off  RndMeth=Floor
  Data Type Conversion3 : DataTypeConversion  OutDataTypeStr=uint8  SampleTime=1e-08  SaturateOnIntegerOverflow=off  RndMeth=Floor
  Data Type Conversion4 : DataTypeConversion  OutDataTypeStr=uint32  SampleTime=1e-08  SaturateOnIntegerOverflow=off  RndMeth=Floor
  CRC : Outport  OutDataTypeStr=uint8  SampleTime=1e-08  InitialOutput=0
  payload : Outport  Port=2  OutDataTypeStr=uint32  SampleTime=1e-08  InitialOutput=0
  error : Outport  Port=3  OutDataTypeStr=boolean  SampleTime=1e-08  InitialOutput=0
  wires:
  Data Type Conversion4/1 -> payload/1
  Data Type Conversion3/1 -> CRC/1
  Data Type Conversion1/1 -> error/1
  Bit Slice4/1 -> Data Type Conversion4/1
  Bit Slice3/1 -> Data Type Conversion3/1
  Bit Slice1/1 -> Data Type Conversion1/1
  DATA/1 -> Bit Slice1/1, Bit Slice3/1, Bit Slice4/1

== system gm_UZ_EnDat/UZ_ENDAT/RESPONSESLICER3X/23BITSLICER/responseslicer ==
  DATA : Inport  OutDataTypeStr=fixdt(0, 64, 0)  PortDimensions=1  SampleTime=1e-08
  Bit Slice1 : hdlsllib/Logic and Bit Operations/Bit Slice  lidx=double(2)  ridx=double(2)
  Bit Slice3 : hdlsllib/Logic and Bit Operations/Bit Slice  lidx=double(29)  ridx=double(25)
  Bit Slice4 : hdlsllib/Logic and Bit Operations/Bit Slice  lidx=double(24)  ridx=double(2)
  Data Type Conversion1 : DataTypeConversion  OutDataTypeStr=boolean  SampleTime=1e-08  SaturateOnIntegerOverflow=off  RndMeth=Floor
  Data Type Conversion3 : DataTypeConversion  OutDataTypeStr=uint8  SampleTime=1e-08  SaturateOnIntegerOverflow=off  RndMeth=Floor
  Data Type Conversion4 : DataTypeConversion  OutDataTypeStr=uint32  SampleTime=1e-08  SaturateOnIntegerOverflow=off  RndMeth=Floor
  CRC : Outport  OutDataTypeStr=uint8  SampleTime=1e-08  InitialOutput=0
  payload : Outport  Port=2  OutDataTypeStr=uint32  SampleTime=1e-08  InitialOutput=0
  error : Outport  Port=3  OutDataTypeStr=boolean  SampleTime=1e-08  InitialOutput=0
  wires:
  DATA/1 -> Bit Slice4/1, Bit Slice3/1, Bit Slice1/1
  Bit Slice1/1 -> Data Type Conversion1/1
  Bit Slice3/1 -> Data Type Conversion3/1
  Bit Slice4/1 -> Data Type Conversion4/1
  Data Type Conversion1/1 -> error/1
  Data Type Conversion3/1 -> CRC/1
  Data Type Conversion4/1 -> payload/1

== system gm_UZ_EnDat/UZ_ENDAT/RESPONSESLICER3X/23BITSLICER/responseslicer1 ==
  DATA : Inport  OutDataTypeStr=fixdt(0, 64, 0)  PortDimensions=1  SampleTime=1e-08
  Bit Slice1 : hdlsllib/Logic and Bit Operations/Bit Slice  lidx=double(2)  ridx=double(2)
  Bit Slice3 : hdlsllib/Logic and Bit Operations/Bit Slice  lidx=double(29)  ridx=double(25)
  Bit Slice4 : hdlsllib/Logic and Bit Operations/Bit Slice  lidx=double(24)  ridx=double(2)
  Data Type Conversion1 : DataTypeConversion  OutDataTypeStr=boolean  SampleTime=1e-08  SaturateOnIntegerOverflow=off  RndMeth=Floor
  Data Type Conversion3 : DataTypeConversion  OutDataTypeStr=uint8  SampleTime=1e-08  SaturateOnIntegerOverflow=off  RndMeth=Floor
  Data Type Conversion4 : DataTypeConversion  OutDataTypeStr=uint32  SampleTime=1e-08  SaturateOnIntegerOverflow=off  RndMeth=Floor
  CRC : Outport  OutDataTypeStr=uint8  SampleTime=1e-08  InitialOutput=0
  payload : Outport  Port=2  OutDataTypeStr=uint32  SampleTime=1e-08  InitialOutput=0
  error : Outport  Port=3  OutDataTypeStr=boolean  SampleTime=1e-08  InitialOutput=0
  wires:
  Data Type Conversion4/1 -> payload/1
  Data Type Conversion3/1 -> CRC/1
  Data Type Conversion1/1 -> error/1
  Bit Slice4/1 -> Data Type Conversion4/1
  Bit Slice3/1 -> Data Type Conversion3/1
  Bit Slice1/1 -> Data Type Conversion1/1
  DATA/1 -> Bit Slice1/1, Bit Slice3/1, Bit Slice4/1

== system gm_UZ_EnDat/UZ_ENDAT/RESPONSESLICER3X/23BITSLICER/responseslicer2 ==
  DATA : Inport  OutDataTypeStr=fixdt(0, 64, 0)  PortDimensions=1  SampleTime=1e-08
  Bit Slice1 : hdlsllib/Logic and Bit Operations/Bit Slice  lidx=double(2)  ridx=double(2)
  Bit Slice3 : hdlsllib/Logic and Bit Operations/Bit Slice  lidx=double(29)  ridx=double(25)
  Bit Slice4 : hdlsllib/Logic and Bit Operations/Bit Slice  lidx=double(24)  ridx=double(2)
  Data Type Conversion1 : DataTypeConversion  OutDataTypeStr=boolean  SampleTime=1e-08  SaturateOnIntegerOverflow=off  RndMeth=Floor
  Data Type Conversion3 : DataTypeConversion  OutDataTypeStr=uint8  SampleTime=1e-08  SaturateOnIntegerOverflow=off  RndMeth=Floor
  Data Type Conversion4 : DataTypeConversion  OutDataTypeStr=uint32  SampleTime=1e-08  SaturateOnIntegerOverflow=off  RndMeth=Floor
  CRC : Outport  OutDataTypeStr=uint8  SampleTime=1e-08  InitialOutput=0
  payload : Outport  Port=2  OutDataTypeStr=uint32  SampleTime=1e-08  InitialOutput=0
  error : Outport  Port=3  OutDataTypeStr=boolean  SampleTime=1e-08  InitialOutput=0
  wires:
  Data Type Conversion4/1 -> payload/1
  Data Type Conversion3/1 -> CRC/1
  Data Type Conversion1/1 -> error/1
  Bit Slice4/1 -> Data Type Conversion4/1
  Bit Slice3/1 -> Data Type Conversion3/1
  Bit Slice1/1 -> Data Type Conversion1/1
  DATA/1 -> Bit Slice1/1, Bit Slice3/1, Bit Slice4/1

== system gm_UZ_EnDat/UZ_ENDAT/RESPONSESLICER3X/25BITSLICER/responseslicer ==
  DATA : Inport  OutDataTypeStr=fixdt(0, 64, 0)  PortDimensions=1  SampleTime=1e-08
  Bit Slice1 : hdlsllib/Logic and Bit Operations/Bit Slice  lidx=double(2)  ridx=double(2)
  Bit Slice3 : hdlsllib/Logic and Bit Operations/Bit Slice  lidx=double(31)  ridx=double(27)
  Bit Slice4 : hdlsllib/Logic and Bit Operations/Bit Slice  lidx=double(26)  ridx=double(2)
  Data Type Conversion1 : DataTypeConversion  OutDataTypeStr=boolean  SampleTime=1e-08  SaturateOnIntegerOverflow=off  RndMeth=Floor
  Data Type Conversion3 : DataTypeConversion  OutDataTypeStr=uint8  SampleTime=1e-08  SaturateOnIntegerOverflow=off  RndMeth=Floor
  Data Type Conversion4 : DataTypeConversion  OutDataTypeStr=uint32  SampleTime=1e-08  SaturateOnIntegerOverflow=off  RndMeth=Floor
  CRC : Outport  OutDataTypeStr=uint8  SampleTime=1e-08  InitialOutput=0
  payload : Outport  Port=2  OutDataTypeStr=uint32  SampleTime=1e-08  InitialOutput=0
  error : Outport  Port=3  OutDataTypeStr=boolean  SampleTime=1e-08  InitialOutput=0
  wires:
  DATA/1 -> Bit Slice4/1, Bit Slice3/1, Bit Slice1/1
  Bit Slice1/1 -> Data Type Conversion1/1
  Bit Slice3/1 -> Data Type Conversion3/1
  Bit Slice4/1 -> Data Type Conversion4/1
  Data Type Conversion1/1 -> error/1
  Data Type Conversion3/1 -> CRC/1
  Data Type Conversion4/1 -> payload/1

== system gm_UZ_EnDat/UZ_ENDAT/RESPONSESLICER3X/25BITSLICER/responseslicer1 ==
  DATA : Inport  OutDataTypeStr=fixdt(0, 64, 0)  PortDimensions=1  SampleTime=1e-08
  Bit Slice1 : hdlsllib/Logic and Bit Operations/Bit Slice  lidx=double(2)  ridx=double(2)
  Bit Slice3 : hdlsllib/Logic and Bit Operations/Bit Slice  lidx=double(31)  ridx=double(27)
  Bit Slice4 : hdlsllib/Logic and Bit Operations/Bit Slice  lidx=double(26)  ridx=double(2)
  Data Type Conversion1 : DataTypeConversion  OutDataTypeStr=boolean  SampleTime=1e-08  SaturateOnIntegerOverflow=off  RndMeth=Floor
  Data Type Conversion3 : DataTypeConversion  OutDataTypeStr=uint8  SampleTime=1e-08  SaturateOnIntegerOverflow=off  RndMeth=Floor
  Data Type Conversion4 : DataTypeConversion  OutDataTypeStr=uint32  SampleTime=1e-08  SaturateOnIntegerOverflow=off  RndMeth=Floor
  CRC : Outport  OutDataTypeStr=uint8  SampleTime=1e-08  InitialOutput=0
  payload : Outport  Port=2  OutDataTypeStr=uint32  SampleTime=1e-08  InitialOutput=0
  error : Outport  Port=3  OutDataTypeStr=boolean  SampleTime=1e-08  InitialOutput=0
  wires:
  Data Type Conversion4/1 -> payload/1
  Data Type Conversion3/1 -> CRC/1
  Data Type Conversion1/1 -> error/1
  Bit Slice4/1 -> Data Type Conversion4/1
  Bit Slice3/1 -> Data Type Conversion3/1
  Bit Slice1/1 -> Data Type Conversion1/1
  DATA/1 -> Bit Slice1/1, Bit Slice3/1, Bit Slice4/1

== system gm_UZ_EnDat/UZ_ENDAT/RESPONSESLICER3X/25BITSLICER/responseslicer2 ==
  DATA : Inport  OutDataTypeStr=fixdt(0, 64, 0)  PortDimensions=1  SampleTime=1e-08
  Bit Slice1 : hdlsllib/Logic and Bit Operations/Bit Slice  lidx=double(2)  ridx=double(2)
  Bit Slice3 : hdlsllib/Logic and Bit Operations/Bit Slice  lidx=double(31)  ridx=double(27)
  Bit Slice4 : hdlsllib/Logic and Bit Operations/Bit Slice  lidx=double(26)  ridx=double(2)
  Data Type Conversion1 : DataTypeConversion  OutDataTypeStr=boolean  SampleTime=1e-08  SaturateOnIntegerOverflow=off  RndMeth=Floor
  Data Type Conversion3 : DataTypeConversion  OutDataTypeStr=uint8  SampleTime=1e-08  SaturateOnIntegerOverflow=off  RndMeth=Floor
  Data Type Conversion4 : DataTypeConversion  OutDataTypeStr=uint32  SampleTime=1e-08  SaturateOnIntegerOverflow=off  RndMeth=Floor
  CRC : Outport  OutDataTypeStr=uint8  SampleTime=1e-08  InitialOutput=0
  payload : Outport  Port=2  OutDataTypeStr=uint32  SampleTime=1e-08  InitialOutput=0
  error : Outport  Port=3  OutDataTypeStr=boolean  SampleTime=1e-08  InitialOutput=0
  wires:
  Data Type Conversion4/1 -> payload/1
  Data Type Conversion3/1 -> CRC/1
  Data Type Conversion1/1 -> error/1
  Bit Slice4/1 -> Data Type Conversion4/1
  Bit Slice3/1 -> Data Type Conversion3/1
  Bit Slice1/1 -> Data Type Conversion1/1
  DATA/1 -> Bit Slice1/1, Bit Slice3/1, Bit Slice4/1

== system gm_UZ_EnDat/UZ_ENDAT/RESPONSESLICER3X/27BITSLICER/responseslicer ==
  DATA : Inport  OutDataTypeStr=fixdt(0, 64, 0)  PortDimensions=1  SampleTime=1e-08
  Bit Slice1 : hdlsllib/Logic and Bit Operations/Bit Slice  lidx=double(2)  ridx=double(2)
  Bit Slice3 : hdlsllib/Logic and Bit Operations/Bit Slice  lidx=double(33)  ridx=double(29)
  Bit Slice4 : hdlsllib/Logic and Bit Operations/Bit Slice  lidx=double(28)  ridx=double(2)
  Data Type Conversion1 : DataTypeConversion  OutDataTypeStr=boolean  SampleTime=1e-08  SaturateOnIntegerOverflow=off  RndMeth=Floor
  Data Type Conversion3 : DataTypeConversion  OutDataTypeStr=uint8  SampleTime=1e-08  SaturateOnIntegerOverflow=off  RndMeth=Floor
  Data Type Conversion4 : DataTypeConversion  OutDataTypeStr=uint32  SampleTime=1e-08  SaturateOnIntegerOverflow=off  RndMeth=Floor
  CRC : Outport  OutDataTypeStr=uint8  SampleTime=1e-08  InitialOutput=0
  payload : Outport  Port=2  OutDataTypeStr=uint32  SampleTime=1e-08  InitialOutput=0
  error : Outport  Port=3  OutDataTypeStr=boolean  SampleTime=1e-08  InitialOutput=0
  wires:
  DATA/1 -> Bit Slice4/1, Bit Slice3/1, Bit Slice1/1
  Bit Slice1/1 -> Data Type Conversion1/1
  Bit Slice3/1 -> Data Type Conversion3/1
  Bit Slice4/1 -> Data Type Conversion4/1
  Data Type Conversion1/1 -> error/1
  Data Type Conversion3/1 -> CRC/1
  Data Type Conversion4/1 -> payload/1

== system gm_UZ_EnDat/UZ_ENDAT/RESPONSESLICER3X/27BITSLICER/responseslicer1 ==
  DATA : Inport  OutDataTypeStr=fixdt(0, 64, 0)  PortDimensions=1  SampleTime=1e-08
  Bit Slice1 : hdlsllib/Logic and Bit Operations/Bit Slice  lidx=double(2)  ridx=double(2)
  Bit Slice3 : hdlsllib/Logic and Bit Operations/Bit Slice  lidx=double(33)  ridx=double(29)
  Bit Slice4 : hdlsllib/Logic and Bit Operations/Bit Slice  lidx=double(28)  ridx=double(2)
  Data Type Conversion1 : DataTypeConversion  OutDataTypeStr=boolean  SampleTime=1e-08  SaturateOnIntegerOverflow=off  RndMeth=Floor
  Data Type Conversion3 : DataTypeConversion  OutDataTypeStr=uint8  SampleTime=1e-08  SaturateOnIntegerOverflow=off  RndMeth=Floor
  Data Type Conversion4 : DataTypeConversion  OutDataTypeStr=uint32  SampleTime=1e-08  SaturateOnIntegerOverflow=off  RndMeth=Floor
  CRC : Outport  OutDataTypeStr=uint8  SampleTime=1e-08  InitialOutput=0
  payload : Outport  Port=2  OutDataTypeStr=uint32  SampleTime=1e-08  InitialOutput=0
  error : Outport  Port=3  OutDataTypeStr=boolean  SampleTime=1e-08  InitialOutput=0
  wires:
  Data Type Conversion4/1 -> payload/1
  Data Type Conversion3/1 -> CRC/1
  Data Type Conversion1/1 -> error/1
  Bit Slice4/1 -> Data Type Conversion4/1
  Bit Slice3/1 -> Data Type Conversion3/1
  Bit Slice1/1 -> Data Type Conversion1/1
  DATA/1 -> Bit Slice1/1, Bit Slice3/1, Bit Slice4/1

== system gm_UZ_EnDat/UZ_ENDAT/RESPONSESLICER3X/27BITSLICER/responseslicer2 ==
  DATA : Inport  OutDataTypeStr=fixdt(0, 64, 0)  PortDimensions=1  SampleTime=1e-08
  Bit Slice1 : hdlsllib/Logic and Bit Operations/Bit Slice  lidx=double(2)  ridx=double(2)
  Bit Slice3 : hdlsllib/Logic and Bit Operations/Bit Slice  lidx=double(33)  ridx=double(29)
  Bit Slice4 : hdlsllib/Logic and Bit Operations/Bit Slice  lidx=double(28)  ridx=double(2)
  Data Type Conversion1 : DataTypeConversion  OutDataTypeStr=boolean  SampleTime=1e-08  SaturateOnIntegerOverflow=off  RndMeth=Floor
  Data Type Conversion3 : DataTypeConversion  OutDataTypeStr=uint8  SampleTime=1e-08  SaturateOnIntegerOverflow=off  RndMeth=Floor
  Data Type Conversion4 : DataTypeConversion  OutDataTypeStr=uint32  SampleTime=1e-08  SaturateOnIntegerOverflow=off  RndMeth=Floor
  CRC : Outport  OutDataTypeStr=uint8  SampleTime=1e-08  InitialOutput=0
  payload : Outport  Port=2  OutDataTypeStr=uint32  SampleTime=1e-08  InitialOutput=0
  error : Outport  Port=3  OutDataTypeStr=boolean  SampleTime=1e-08  InitialOutput=0
  wires:
  Data Type Conversion4/1 -> payload/1
  Data Type Conversion3/1 -> CRC/1
  Data Type Conversion1/1 -> error/1
  Bit Slice4/1 -> Data Type Conversion4/1
  Bit Slice3/1 -> Data Type Conversion3/1
  Bit Slice1/1 -> Data Type Conversion1/1
  DATA/1 -> Bit Slice1/1, Bit Slice3/1, Bit Slice4/1
